simulink model "FullSystem"  (R2024a)
settings: Solver=VariableStepAuto  StartTime=0.0  StopTime=14*3600  RelTol=1e-3
undefined symbols (not defined in the file or in its folder): Beta, D_eq_Linear, GearRatio, I_eq_NonLinear, I_motor, I_Pole, k_b, k_t, L_Motor, Length_Panel, Mass_Panel, R_Motor, StartingPosition, TF_Denom_2, TF_Denom_3, TF_Num_2, TF_Num_3, Thickness_Panel, Width_Panel
libraries: simulink x14, slpidlib x3, slctrl_linear x1
settings Model: Creator=jonat  LastModifiedBy=jonat
settings DataIOCC: ExternalInput=[sunTime,sunPos]  LoadExternalInput=on

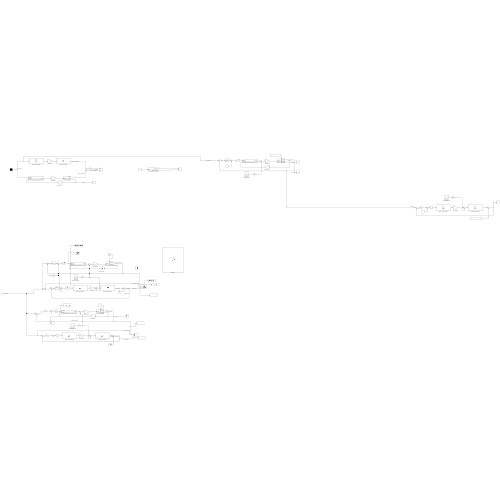
[thumbnail: Simulink's stored preview of the top-level diagram]
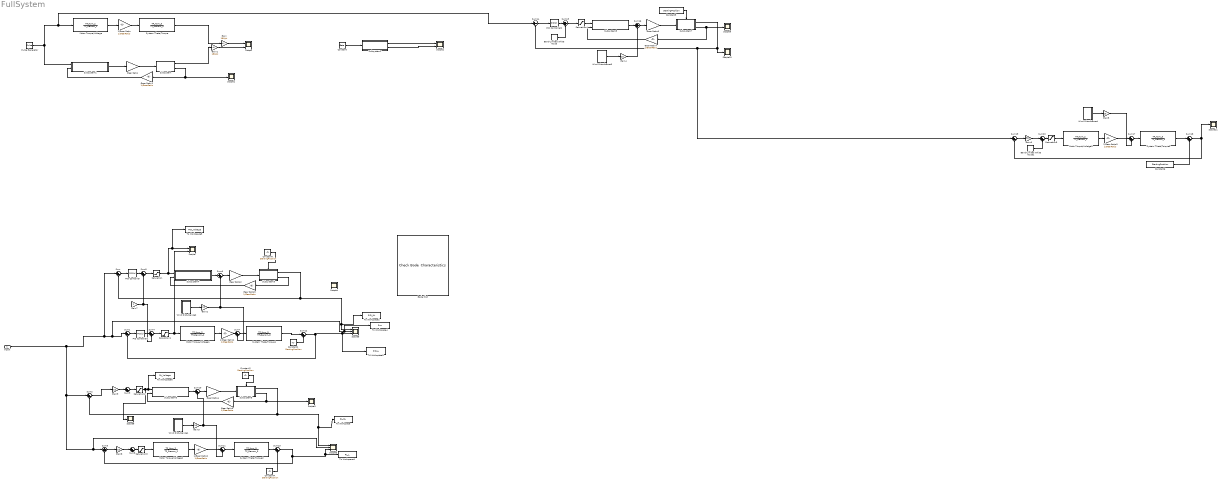
== system FullSystem ==
  Inport : Inport
  1/Gear Ratio{,1..3} (4 alike) : Gain  Gain=1/GearRatio
  Band-Limited White Noise : simulink/Sources/Band-Limited White Noise  Cov=[0.1]  Ts=0.1  seed=[23341]
  Band-Limited White Noise1 : simulink/Sources/Band-Limited White Noise  Cov=[0.1]  Ts=0.1  seed=[23341]
  Bode Plot : slctrl_linear/Check Bode  Characteristics  InstantiateOnLoad=on  SaveOperatingPoints=off  LinearizationIOs={'/PID Controller', 1, 'in', 'off', '';'/Subsystem3', 1, 'out', 'off', ''}  LinearizeAt=SnapshotTimes  SnapshotTimes=[0]  TriggerType=rising  SampleTime=auto  RateConversionMethod=zoh  PreWarpFreq=10  UseExactDelayModel=off  UseFullBlockNameLabels=off  UseBusSignalLabels=off  enabled=on  stopWhenAssertionFail=off  export=off  ViewDlgPos=[345 171 1226 663]  OpenViewOnLoad=off  LaunchViewOnOpen=on  FrequencyUnits=rad/s  MagnitudeUnits=dB  PhaseUnits=deg  TimeUnits=seconds  EnableUpperBound=off  UpperBoundFrequencies=[]  UpperBoundMagnitudes=[]  EnableLowerBound=off  LowerBoundFrequencies=[]  LowerBoundMagnitudes=[]
      settings: LibrarySourceBlock=slctrlblks/Linear Analysis Plots/Bode Plot  SaveToWorkspace=off  SaveName=sys
  Constant : Constant  Value=Beta
  Constant{1..6} (6 alike) : Constant  Value=StartingPosition
  Gain : Gain  Gain=180/pi
  Gain1 : Gain  Gain=180/pi
  Gain{2..5} (4 alike) : Gain  Gain=10
  Gain6 : Gain  Gain=910
  Gain7 : Gain
  Gain8 : Gain  Gain=910
  Gain9 : Gain  Gain=910
  Gear Ratio{,2,4,6} (4 alike) : Gain  Gain=GearRatio
  Gear Ratio{1,3,5,7} (4 alike) : Gain  Gain=1/GearRatio
  Motor Torque/Voltage{,1..3} (4 alike) : TransferFcn  Numerator=TF_Num_2  Denominator=TF_Denom_2
  PID Controller : slpidlib/PID Controller  Controller=PID  Form=Parallel  TimeDomain=Continuous-time  UseExternalTs=off  SampleTime=-1  IntegratorMethod=Forward Euler  FilterMethod=Forward Euler  ControllerParametersSource=internal  P=900  I=2  UseKiTs=off  D=0.1  UseExternalDerivativeSource=off  N=100  UseFilter=on  TunerSelectOption=Transfer Function Based (PID Tuner App)  InitialConditionSource=internal  InitialConditionForIntegrator=0  InitialConditionForFilter=0  DifferentiatorICPrevScaledInput=0  ExternalReset=none  TrackingMode=off  Kt=1  LimitOutput=off  SatLimitsSource=internal  UpperSaturationLimit=inf  LowerSaturationLimit=-inf  LinearizeAsGain=on  AntiWindupMode=none  Kb=1  LimitIntegrator=off  UpperIntegratorSaturationLimit=inf  LowerIntegratorSaturationLimit=-inf  POutMin=[]  POutMax=[]  IOutMin=[]  IOutMax=[]  DOutMin=[]  DOutMax=[]  NOutMin=[]  NOutMax=[]  SumOutMin=[]  SumOutMax=[]  SaturationOutMin=[]  SaturationOutMax=[]  PParamMin=[]  PParamMax=[]  IParamMin=[]  IParamMax=[]  DParamMin=[]  DParamMax=[]  NParamMin=[]  NParamMax=[]  KbParamMin=[]  KbParamMax=[]  KtParamMin=[]  KtParamMax=[]  KbOutMin=[]  KbOutMax=[]  KtOutMin=[]  KtOutMax=[]  IntegratorOutMin=[]  IntegratorOutMax=[]  FilterOutMin=[]  FilterOutMax=[]  SumI1OutMin=[]  SumI1OutMax=[]  SumI2OutMin=[]  SumI2OutMax=[]  SumI3OutMin=[]  SumI3OutMax=[]  SumI4OutMin=[]  SumI4OutMax=[]  SumDOutMin=[]  SumDOutMax=[]  DifferentiatorOutMin=[]  DifferentiatorOutMax=[]  FilterDiffOutCoefMin=[]  FilterDiffOutCoefMax=[]  ReciprocalOutMin=[]  ReciprocalOutMax=[]  SumDenOutMin=[]  SumDenOutMax=[]  SumNumOutMin=[]  SumNumOutMax=[]  DivideOutMin=[]  DivideOutMax=[]  UdiffTsProdOutMin=[]  UdiffTsProdOutMax=[]  NTsProdOutMin=[]  NTsProdOutMax=[]  UintegralTsProdOutMin=[]  UintegralTsProdOutMax=[]  UngainTsProdOutMin=[]  UngainTsProdOutMax=[]  ClampingZeroOutDataTypeStr=Inherit: Inherit via back propagation  ClampingZeroOutMin=[]  ClampingZeroOutMax=[]  FilterDenConstantOutDataTypeStr=Inherit: Inherit via back propagation  FilterDenConstantOutMin=[]  FilterDenConstantOutMax=[]  PCopyOutDataTypeStr=Inherit: Inherit via back propagation  PCopyOutMin=[]  PCopyOutMax=[]  NCopyOutDataTypeStr=Inherit: Inherit via back propagation  NCopyOutMin=[]  NCopyOutMax=[]  IntegratorContinuousStateAttributes=''  IntegratorStateMustResolveToSignalObject=off  IntegratorRTWStateStorageClass=Auto  FilterContinuousStateAttributes=''  FilterStateMustResolveToSignalObject=off  FilterRTWStateStorageClass=Auto  ParallelPVariant=InternalParameters  IdealPVariant=Disabled  IVariant=InternalParameters  DVariant=InternalParameters  IntegratorVariant=Continuous  SatVariant=Disabled  AWVariant=Passthrough  PCopyVariant=Disabled  TRVariant=Disabled  FdbkBlocksVariant=Forward  IdealPFdbkVariant=Disabled  SatFdbkVariant=Disabled  DerivativeFilterVariant=ContFilter  NVariant=InternalParameters  NCopyVariant=Disabled  FilterICVariant=InternalICsFilter  IntegratorICVariant=InternalICs  ExternalResetVariant=Disabled  TRSumVariant=Passthrough  SumFdbkVariant=Disabled  SumVariant=Sum_PID  TsampFilterVariant=InternalTs  TsampNgainVariant=Passthrough  TsampIntegralVariant=Disabled_SignalSpec  ExternalSaturationOutDataTypeStr=Inherit: Same as second input  DerivativeSourceVariant=ErrorSignal
  PID Controller1 : slpidlib/PID Controller  Controller=PID  Form=Parallel  TimeDomain=Continuous-time  UseExternalTs=off  SampleTime=-1  IntegratorMethod=Forward Euler  FilterMethod=Forward Euler  ControllerParametersSource=internal  P=900  I=2  UseKiTs=off  D=0.1  UseExternalDerivativeSource=off  N=2.09794311620465  UseFilter=on  TunerSelectOption=Transfer Function Based (PID Tuner App)  InitialConditionSource=internal  InitialConditionForIntegrator=0  InitialConditionForFilter=0  DifferentiatorICPrevScaledInput=0  ExternalReset=none  TrackingMode=off  Kt=1  LimitOutput=off  SatLimitsSource=internal  UpperSaturationLimit=inf  LowerSaturationLimit=-inf  LinearizeAsGain=on  AntiWindupMode=none  Kb=1  LimitIntegrator=off  UpperIntegratorSaturationLimit=inf  LowerIntegratorSaturationLimit=-inf  POutMin=[]  POutMax=[]  IOutMin=[]  IOutMax=[]  DOutMin=[]  DOutMax=[]  NOutMin=[]  NOutMax=[]  SumOutMin=[]  SumOutMax=[]  SaturationOutMin=[]  SaturationOutMax=[]  PParamMin=[]  PParamMax=[]  IParamMin=[]  IParamMax=[]  DParamMin=[]  DParamMax=[]  NParamMin=[]  NParamMax=[]  KbParamMin=[]  KbParamMax=[]  KtParamMin=[]  KtParamMax=[]  KbOutMin=[]  KbOutMax=[]  KtOutMin=[]  KtOutMax=[]  IntegratorOutMin=[]  IntegratorOutMax=[]  FilterOutMin=[]  FilterOutMax=[]  SumI1OutMin=[]  SumI1OutMax=[]  SumI2OutMin=[]  SumI2OutMax=[]  SumI3OutMin=[]  SumI3OutMax=[]  SumI4OutMin=[]  SumI4OutMax=[]  SumDOutMin=[]  SumDOutMax=[]  DifferentiatorOutMin=[]  DifferentiatorOutMax=[]  FilterDiffOutCoefMin=[]  FilterDiffOutCoefMax=[]  ReciprocalOutMin=[]  ReciprocalOutMax=[]  SumDenOutMin=[]  SumDenOutMax=[]  SumNumOutMin=[]  SumNumOutMax=[]  DivideOutMin=[]  DivideOutMax=[]  UdiffTsProdOutMin=[]  UdiffTsProdOutMax=[]  NTsProdOutMin=[]  NTsProdOutMax=[]  UintegralTsProdOutMin=[]  UintegralTsProdOutMax=[]  UngainTsProdOutMin=[]  UngainTsProdOutMax=[]  ClampingZeroOutDataTypeStr=Inherit: Inherit via back propagation  ClampingZeroOutMin=[]  ClampingZeroOutMax=[]  FilterDenConstantOutDataTypeStr=Inherit: Inherit via back propagation  FilterDenConstantOutMin=[]  FilterDenConstantOutMax=[]  PCopyOutDataTypeStr=Inherit: Inherit via back propagation  PCopyOutMin=[]  PCopyOutMax=[]  NCopyOutDataTypeStr=Inherit: Inherit via back propagation  NCopyOutMin=[]  NCopyOutMax=[]  IntegratorContinuousStateAttributes=''  IntegratorStateMustResolveToSignalObject=off  IntegratorRTWStateStorageClass=Auto  FilterContinuousStateAttributes=''  FilterStateMustResolveToSignalObject=off  FilterRTWStateStorageClass=Auto  ParallelPVariant=InternalParameters  IdealPVariant=Disabled  IVariant=InternalParameters  DVariant=InternalParameters  IntegratorVariant=Continuous  SatVariant=Disabled  AWVariant=Passthrough  PCopyVariant=Disabled  TRVariant=Disabled  FdbkBlocksVariant=Forward  IdealPFdbkVariant=Disabled  SatFdbkVariant=Disabled  DerivativeFilterVariant=ContFilter  NVariant=InternalParameters  NCopyVariant=Disabled  FilterICVariant=InternalICsFilter  IntegratorICVariant=InternalICs  ExternalResetVariant=Disabled  TRSumVariant=Passthrough  SumFdbkVariant=Disabled  SumVariant=Sum_PID  TsampFilterVariant=InternalTs  TsampNgainVariant=Passthrough  TsampIntegralVariant=Disabled_SignalSpec  ExternalSaturationOutDataTypeStr=Inherit: Same as second input  DerivativeSourceVariant=ErrorSignal
  PID Controller2 : slpidlib/PID Controller  Controller=PID  Form=Parallel  TimeDomain=Continuous-time  UseExternalTs=off  SampleTime=-1  IntegratorMethod=Forward Euler  FilterMethod=Forward Euler  ControllerParametersSource=internal  P=900  I=2  UseKiTs=off  D=0.1  UseExternalDerivativeSource=off  N=100  UseFilter=on  TunerSelectOption=Transfer Function Based (PID Tuner App)  InitialConditionSource=internal  InitialConditionForIntegrator=0  InitialConditionForFilter=0  DifferentiatorICPrevScaledInput=0  ExternalReset=none  TrackingMode=off  Kt=1  LimitOutput=off  SatLimitsSource=internal  UpperSaturationLimit=inf  LowerSaturationLimit=-inf  LinearizeAsGain=on  AntiWindupMode=none  Kb=1  LimitIntegrator=off  UpperIntegratorSaturationLimit=inf  LowerIntegratorSaturationLimit=-inf  POutMin=[]  POutMax=[]  IOutMin=[]  IOutMax=[]  DOutMin=[]  DOutMax=[]  NOutMin=[]  NOutMax=[]  SumOutMin=[]  SumOutMax=[]  SaturationOutMin=[]  SaturationOutMax=[]  PParamMin=[]  PParamMax=[]  IParamMin=[]  IParamMax=[]  DParamMin=[]  DParamMax=[]  NParamMin=[]  NParamMax=[]  KbParamMin=[]  KbParamMax=[]  KtParamMin=[]  KtParamMax=[]  KbOutMin=[]  KbOutMax=[]  KtOutMin=[]  KtOutMax=[]  IntegratorOutMin=[]  IntegratorOutMax=[]  FilterOutMin=[]  FilterOutMax=[]  SumI1OutMin=[]  SumI1OutMax=[]  SumI2OutMin=[]  SumI2OutMax=[]  SumI3OutMin=[]  SumI3OutMax=[]  SumI4OutMin=[]  SumI4OutMax=[]  SumDOutMin=[]  SumDOutMax=[]  DifferentiatorOutMin=[]  DifferentiatorOutMax=[]  FilterDiffOutCoefMin=[]  FilterDiffOutCoefMax=[]  ReciprocalOutMin=[]  ReciprocalOutMax=[]  SumDenOutMin=[]  SumDenOutMax=[]  SumNumOutMin=[]  SumNumOutMax=[]  DivideOutMin=[]  DivideOutMax=[]  UdiffTsProdOutMin=[]  UdiffTsProdOutMax=[]  NTsProdOutMin=[]  NTsProdOutMax=[]  UintegralTsProdOutMin=[]  UintegralTsProdOutMax=[]  UngainTsProdOutMin=[]  UngainTsProdOutMax=[]  ClampingZeroOutDataTypeStr=Inherit: Inherit via back propagation  ClampingZeroOutMin=[]  ClampingZeroOutMax=[]  FilterDenConstantOutDataTypeStr=Inherit: Inherit via back propagation  FilterDenConstantOutMin=[]  FilterDenConstantOutMax=[]  PCopyOutDataTypeStr=Inherit: Inherit via back propagation  PCopyOutMin=[]  PCopyOutMax=[]  NCopyOutDataTypeStr=Inherit: Inherit via back propagation  NCopyOutMin=[]  NCopyOutMax=[]  IntegratorContinuousStateAttributes=''  IntegratorStateMustResolveToSignalObject=off  IntegratorRTWStateStorageClass=Auto  FilterContinuousStateAttributes=''  FilterStateMustResolveToSignalObject=off  FilterRTWStateStorageClass=Auto  ParallelPVariant=InternalParameters  IdealPVariant=Disabled  IVariant=InternalParameters  DVariant=InternalParameters  IntegratorVariant=Continuous  SatVariant=Disabled  AWVariant=Passthrough  PCopyVariant=Disabled  TRVariant=Disabled  FdbkBlocksVariant=Forward  IdealPFdbkVariant=Disabled  SatFdbkVariant=Disabled  DerivativeFilterVariant=ContFilter  NVariant=InternalParameters  NCopyVariant=Disabled  FilterICVariant=InternalICsFilter  IntegratorICVariant=InternalICs  ExternalResetVariant=Disabled  TRSumVariant=Passthrough  SumFdbkVariant=Disabled  SumVariant=Sum_PID  TsampFilterVariant=InternalTs  TsampNgainVariant=Passthrough  TsampIntegralVariant=Disabled_SignalSpec  ExternalSaturationOutDataTypeStr=Inherit: Same as second input  DerivativeSourceVariant=ErrorSignal
  Pulse Generator : DiscretePulseGenerator  PulseType=Time based  Amplitude=5  Period=400
  Saturation{,1..5} (6 alike) : Saturate  UpperLimit=220  LowerLimit=-220
  Scope : Scope  NumInputPorts=2
  Scope{1,3..4,8..11} (7 alike) : Scope
  Scope2 : Scope  NumInputPorts=2
  Scope5 : Scope  NumInputPorts=3
  Scope6 : Scope  NumInputPorts=3
  Scope7 : Scope  NumInputPorts=2
  Subsystem : Subsystem
  Subsystem1 : Subsystem
  Subsystem2 : Subsystem
  Subsystem3 : Subsystem
      settings: PortSchema="{\"entries\":[{\"content\":{\"sides\":[{\"content\":{\"connectorIds\":[\"In1\"]},\"type\":\"ConnectorPlacement.EquallySpacedRectSide\",\"uuid\":\"8ea1f8af-770d-4a24-b012-ba6e01ad0303\"},{\"content\":{\"connectorIds\":[\"Out1\",\"Out2\"],\"side\":\"RIGHT\"},\"type\":\"ConnectorPlacement.EquallySpacedRectSide\",\"uuid\":\"5c008235-f776-4735-b061-be577f1b76a0\"},{\"content\":{\"connectorIds\":[\"In2\"],\"side\":\"TOP\"},\"type\":\"ConnectorPlacement.EquallySpacedRectSide\",\"uuid\":\"8e8587eb-de19-4631-a42c-bfa0ae223d11\"}]},\"type\":\"ConnectorPlacement.EquallySpacedConnector\",\"uuid\":\"de8c275b-bedc-409d-bb08-97ede13c9c40\"}],\"packageUris\":[\"http://schema.mathworks.com/mf0/Connector/R2020b\"],\"version\":\"1.0\"}"
  Subsystem4 : Subsystem
  Subsystem5 : Subsystem
      settings: PortSchema="{\"entries\":[{\"content\":{\"sides\":[{\"content\":{\"connectorIds\":[\"In1\"]},\"type\":\"ConnectorPlacement.EquallySpacedRectSide\",\"uuid\":\"8ea1f8af-770d-4a24-b012-ba6e01ad0303\"},{\"content\":{\"connectorIds\":[\"Out1\",\"Out2\"],\"side\":\"RIGHT\"},\"type\":\"ConnectorPlacement.EquallySpacedRectSide\",\"uuid\":\"5c008235-f776-4735-b061-be577f1b76a0\"},{\"content\":{\"connectorIds\":[\"In2\"],\"side\":\"TOP\"},\"type\":\"ConnectorPlacement.EquallySpacedRectSide\",\"uuid\":\"8e8587eb-de19-4631-a42c-bfa0ae223d11\"}]},\"type\":\"ConnectorPlacement.EquallySpacedConnector\",\"uuid\":\"de8c275b-bedc-409d-bb08-97ede13c9c40\"}],\"packageUris\":[\"http://schema.mathworks.com/mf0/Connector/R2020b\"],\"version\":\"1.0\"}"
  Subsystem6 : Subsystem
  Subsystem7 : Subsystem
      settings: PortSchema="{\"entries\":[{\"content\":{\"sides\":[{\"content\":{\"connectorIds\":[\"In1\"]},\"type\":\"ConnectorPlacement.EquallySpacedRectSide\",\"uuid\":\"8ea1f8af-770d-4a24-b012-ba6e01ad0303\"},{\"content\":{\"connectorIds\":[\"Out1\",\"Out2\"],\"side\":\"RIGHT\"},\"type\":\"ConnectorPlacement.EquallySpacedRectSide\",\"uuid\":\"5c008235-f776-4735-b061-be577f1b76a0\"},{\"content\":{\"connectorIds\":[\"In2\"],\"side\":\"TOP\"},\"type\":\"ConnectorPlacement.EquallySpacedRectSide\",\"uuid\":\"8e8587eb-de19-4631-a42c-bfa0ae223d11\"}]},\"type\":\"ConnectorPlacement.EquallySpacedConnector\",\"uuid\":\"de8c275b-bedc-409d-bb08-97ede13c9c40\"}],\"packageUris\":[\"http://schema.mathworks.com/mf0/Connector/R2020b\"],\"version\":\"1.0\"}"
  Subsystem8 : Subsystem
  Sum{,1..3,14,19} (6 alike) : Sum  Inputs=|+-
  Sum{4..13,15..18,20} (15 alike) : Sum  Inputs=|++
  System Theta/Torque{,1..3} (4 alike) : TransferFcn  Numerator=TF_Num_3  Denominator=TF_Denom_3
  To Workspace : ToWorkspace  VariableName=RL_NL  SampleTime=-1
  To Workspace1 : ToWorkspace  VariableName=RL_L  SampleTime=-1
  To Workspace2 : ToWorkspace  VariableName=PID_NL  SampleTime=-1
  To Workspace3 : ToWorkspace  VariableName=PID_L  SampleTime=-1
  To Workspace4 : ToWorkspace  VariableName=Sun  SampleTime=-1
  To Workspace5 : ToWorkspace  VariableName=PID_Voltage  SampleTime=-1
  To Workspace6 : ToWorkspace  VariableName=RL_Voltage  SampleTime=-1
  Wind Disturbance1 : Subsystem
  Wind Disturbance2 : Subsystem
  Wind Disturbance3 : Subsystem
  Wind Disturbance4 : Subsystem
  wires:
  Subsystem/1(Position) -> Gain1/1  "Position Non-Linear"
  Subsystem/2(Velocity) -> Gear Ratio1/1, Scope1/1  "Velocity"
  Subsystem1/1(Torque) -> Gear Ratio/1
  Gear Ratio/1 -> Subsystem/1(Torque)
  1/Gear Ratio/1 -> System Theta/Torque/1
  Motor Torque/Voltage/1 -> 1/Gear Ratio/1
  System Theta/Torque/1 -> Gain/1  "Position Linear Model"
  Gear Ratio1/1 -> Subsystem1/2(Velocity)
  Constant/1 -> Subsystem2/1(Beta)
  Subsystem2/1(MOI Linear) -> Scope2/1
  Subsystem2/2(MOI Non Linear) -> Scope2/2
  Gain/1 -> Scope/1  "Linear Model"
  Gain1/1 -> Scope/2  "Non-Linear Model"
  Subsystem3/1(Position) -> Scope5/1, To Workspace2/1, Sum/2  "Position Non-Linear"
  Subsystem4/1(Torque) -> Sum6/1
  Gear Ratio2/1 -> Subsystem3/1(Torque)
  Subsystem3/2(Velocity) -> Gear Ratio3/1  "Velocity"
  Gear Ratio3/1 -> Subsystem4/2(Velocity)
  Sum/1 -> PID Controller/1  "Error"
  PID Controller/1 -> Sum5/1
  Motor Torque/Voltage1/1 -> 1/Gear Ratio1/1
  1/Gear Ratio1/1 -> Sum7/1
  PID Controller1/1 -> Sum4/1
  Sum1/1 -> PID Controller1/1  "Error"
  Sum12/1 -> Sum1/2, To Workspace3/1, Scope5/3  "Linear Model"
  1/Gear Ratio2/1 -> Sum11/1
  Motor Torque/Voltage2/1 -> 1/Gear Ratio2/1
  Subsystem6/1(Torque) -> Sum10/1
  Sum2/1 -> Gain9/1  "Error"
  Gear Ratio5/1 -> Subsystem6/2(Velocity)
  Gear Ratio4/1 -> Subsystem5/1(Torque)
  Sum3/1 -> Gain8/1  "Error"
  Subsystem5/2(Velocity) -> Gear Ratio5/1, Scope3/1  "Velocity"
  Subsystem5/1(Position) -> Sum2/2, Scope6/1, To Workspace/1  "Position Non-Linear"
  Sum4/1 -> Saturation1/1
  Sum13/1 -> To Workspace1/1, Scope6/3, Sum3/2  "Linear Model"
  Gain8/1 -> Sum8/1
  Gain9/1 -> Sum9/1
  Inport/1 -> Sum2/1, Scope6/2, Sum3/1, Sum/1, To Workspace4/1, Scope5/2, Sum1/1  "Sun Positon"
  Sum6/1 -> Gear Ratio2/1
  Sum7/1 -> System Theta/Torque1/1
  Sum9/1 -> Saturation2/1
  Sum10/1 -> Gear Ratio4/1
  Sum11/1 -> System Theta/Torque2/1
  Gain3/1 -> Sum11/2, Sum10/2
  Gain2/1 -> Sum7/2, Sum6/2
  Wind Disturbance1/1(Out1) -> Gain3/1
  System Theta/Torque1/1 -> Sum12/1  "Linear Model"
  Constant1/1 -> Sum12/2
  Sum5/1 -> Saturation/1
  Saturation/1 -> Subsystem4/1(Voltage), To Workspace5/1, Scope7/1
  Constant2/1 -> Subsystem3/2(StartPos)
  Constant3/1 -> Subsystem5/2(StartPosRL)
  System Theta/Torque2/1 -> Sum13/1  "Linear Model"
  Constant4/1 -> Sum13/2
  Saturation1/1 -> Scope7/2, Motor Torque/Voltage1/1
  Saturation2/1 -> Scope8/1, To Workspace6/1, Subsystem6/1(Voltage)
  Sum8/1 -> Saturation3/1
  Saturation3/1 -> Motor Torque/Voltage2/1
  Gain7/1 -> Sum4/2, Sum5/2
  Band-Limited White Noise/1 -> Sum15/2
  Saturation4/1 -> Subsystem8/1(Voltage)
  Subsystem7/2(Velocity) -> Gear Ratio7/1, Scope9/1  "Velocity"
  Pulse Generator/1 -> Sum14/1, Motor Torque/Voltage/1, Subsystem1/1(Voltage)  "Sun Positon"
  Constant5/1 -> Subsystem7/2(StartPos)
  Gain4/1 -> Sum16/2
  Sum14/1 -> PID Controller2/1  "Error"
  Sum15/1 -> Saturation4/1
  Gear Ratio6/1 -> Subsystem7/1(Torque)
  Wind Disturbance3/1(Out1) -> Gain4/1
  Sum16/1 -> Gear Ratio6/1
  Gear Ratio7/1 -> Subsystem8/2(Velocity)
  PID Controller2/1 -> Sum15/1
  Subsystem8/1(Torque) -> Sum16/1
  System Theta/Torque3/1 -> Sum18/1
  Sum20/1 -> Saturation5/1
  Saturation5/1 -> Motor Torque/Voltage3/1
  Constant6/1 -> Sum18/2
  Sum17/1 -> System Theta/Torque3/1
  Sum18/1 -> Sum19/2, Scope11/1
  Gain5/1 -> Sum17/2
  Gain6/1 -> Sum20/1
  Subsystem7/1(Position) -> Sum19/1, Sum14/2, Scope10/1  "Sun Positon"
  1/Gear Ratio3/1 -> Sum17/1
  Motor Torque/Voltage3/1 -> 1/Gear Ratio3/1
  Sum19/1 -> Gain6/1  "Error"
  Wind Disturbance4/1(Out1) -> Gain5/1
  Band-Limited White Noise1/1 -> Sum20/2
  ? -> Gain7/1
  Wind Disturbance2/1(Out1) -> Gain2/1

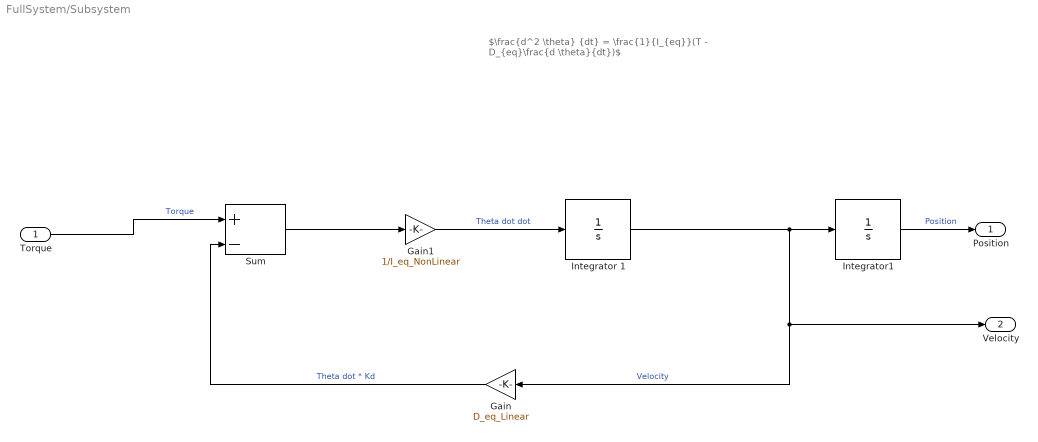
== system FullSystem/Subsystem ==
  note: $\frac{d^2 \theta} {dt} = \frac{1}{I_{eq}}(T - D_{eq}\frac{d \theta}{dt})$
  Torque : Inport
  Gain : Gain  Gain=D_eq_Linear
  Gain1 : Gain  Gain=1/I_eq_NonLinear
  Integrator 1 : Integrator
  Integrator1 : Integrator
  Sum : Sum  Inputs=|+-
  Position : Outport
  Velocity : Outport  Port=2
  wires:
  Sum/1 -> Gain1/1
  Integrator1/1 -> Position/1  "Position"
  Gain1/1 -> Integrator 1/1  "Theta dot dot"
  Integrator 1/1 -> Velocity/1, Gain/1, Integrator1/1  "Velocity"
  Torque/1 -> Sum/1  "Torque"
  Gain/1 -> Sum/2  "Theta dot * Kd"

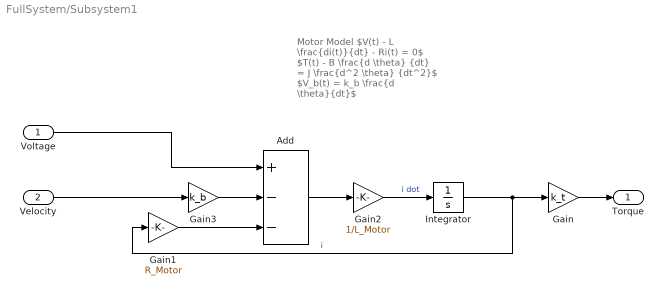
== system FullSystem/Subsystem1 ==
  note: Motor Model
      | $V(t) - L \frac{di(t)}{dt} - Ri(t) = 0$
      | $T(t) - B \frac{d \theta} {dt} = J \frac{d^2 \theta} {dt^2}$
      | $V_b(t) = k_b \frac{d \theta}{dt}$
  Voltage : Inport
  Velocity : Inport  Port=2
  Add : Sum  Inputs=+--
  Gain : Gain  Gain=k_t
  Gain1 : Gain  Gain=R_Motor
  Gain2 : Gain  Gain=1/L_Motor
  Gain3 : Gain  Gain=k_b
  Integrator : Integrator
  Torque : Outport
  wires:
  Integrator/1 -> Gain/1, Gain1/1  "i"
  Add/1 -> Gain2/1
  Gain3/1 -> Add/2
  Velocity/1 -> Gain3/1
  Voltage/1 -> Add/1
  Gain/1 -> Torque/1
  Gain2/1 -> Integrator/1  "i dot"
  Gain1/1 -> Add/3

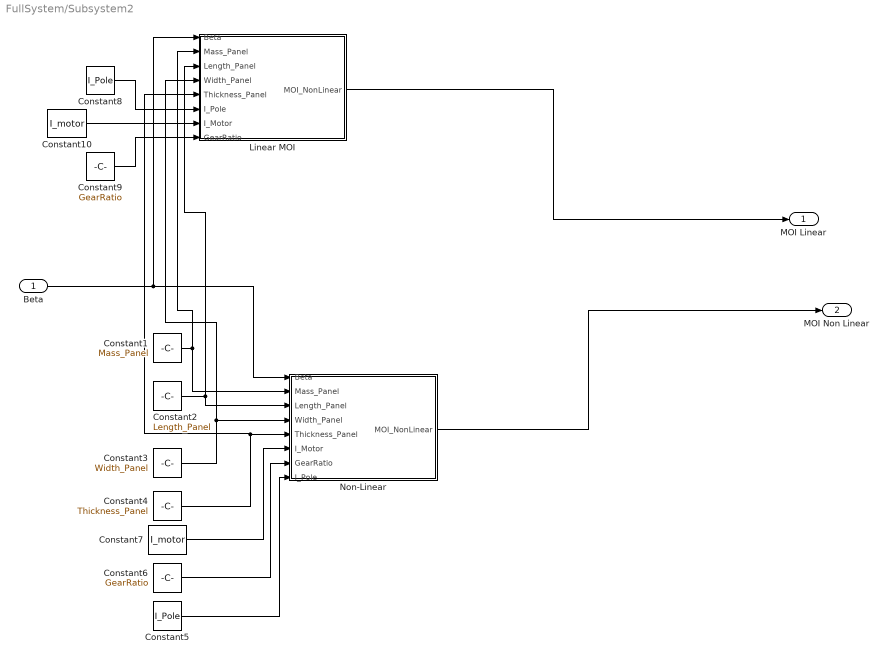
== system FullSystem/Subsystem2 ==
  Beta : Inport
  Constant1 : Constant  Value=Mass_Panel
  Constant10 : Constant  Value=I_motor
  Constant2 : Constant  Value=Length_Panel
  Constant3 : Constant  Value=Width_Panel
  Constant4 : Constant  Value=Thickness_Panel
  Constant5 : Constant  Value=I_Pole
  Constant6 : Constant  Value=GearRatio
  Constant7 : Constant  Value=I_motor
  Constant8 : Constant  Value=I_Pole
  Constant9 : Constant  Value=GearRatio
  Linear MOI : MATLAB Function  TreatAsAtomicUnit=on
  Non-Linear : MATLAB Function  TreatAsAtomicUnit=on
  MOI Linear : Outport
  MOI Non Linear : Outport  Port=2
  wires:
  Constant2/1 -> Linear MOI/3(Length_Panel), Non-Linear/3(Length_Panel)
  Constant6/1 -> Non-Linear/7(GearRatio)
  Constant8/1 -> Linear MOI/6(I_Pole)
  Constant3/1 -> Non-Linear/4(Width_Panel), Linear MOI/4(Width_Panel)
  Constant4/1 -> Non-Linear/5(Thickness_Panel), Linear MOI/5(Thickness_Panel)
  Beta/1 -> Linear MOI/1(Beta), Non-Linear/1(Beta)
  Constant1/1 -> Linear MOI/2(Mass_Panel), Non-Linear/2(Mass_Panel)
  Constant10/1 -> Linear MOI/7(I_Motor)
  Constant7/1 -> Non-Linear/6(I_Motor)
  Constant9/1 -> Linear MOI/8(GearRatio)
  Constant5/1 -> Non-Linear/8(I_Pole)
  Non-Linear/1(MOI_NonLinear) -> MOI Non Linear/1
  Linear MOI/1(MOI_NonLinear) -> MOI Linear/1

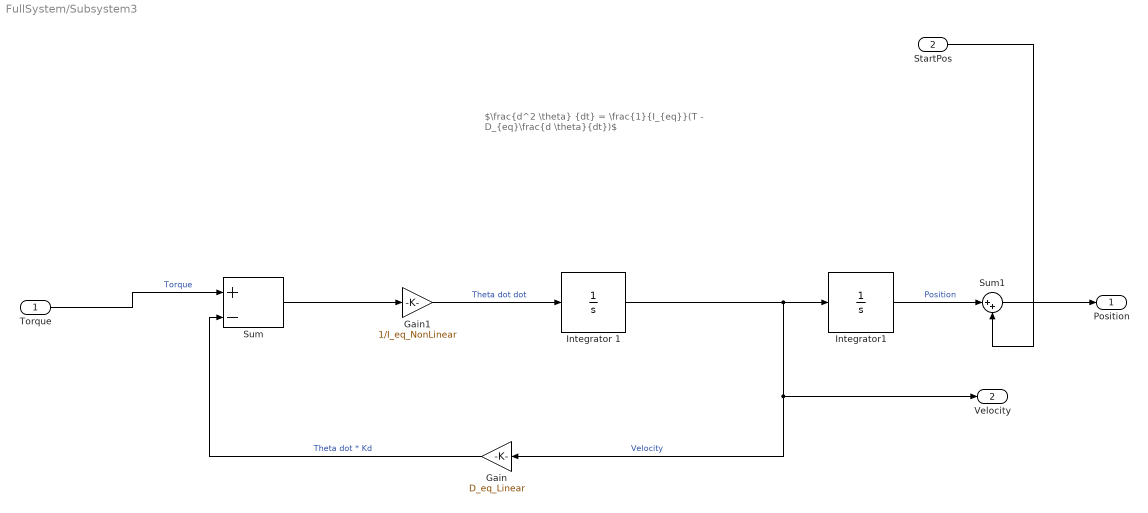
== system FullSystem/Subsystem3 ==
  note: $\frac{d^2 \theta} {dt} = \frac{1}{I_{eq}}(T - D_{eq}\frac{d \theta}{dt})$
  Torque : Inport
  StartPos : Inport  Port=2
  Gain : Gain  Gain=D_eq_Linear
  Gain1 : Gain  Gain=1/I_eq_NonLinear
  Integrator 1 : Integrator
  Integrator1 : Integrator
  Sum : Sum  Inputs=|+-
  Sum1 : Sum  Inputs=|++
  Position : Outport
  Velocity : Outport  Port=2
  wires:
  Sum/1 -> Gain1/1
  Integrator1/1 -> Sum1/1  "Position"
  Gain1/1 -> Integrator 1/1  "Theta dot dot"
  Integrator 1/1 -> Velocity/1, Gain/1, Integrator1/1  "Velocity"
  Torque/1 -> Sum/1  "Torque"
  Gain/1 -> Sum/2  "Theta dot * Kd"
  Sum1/1 -> Position/1
  StartPos/1 -> Sum1/2

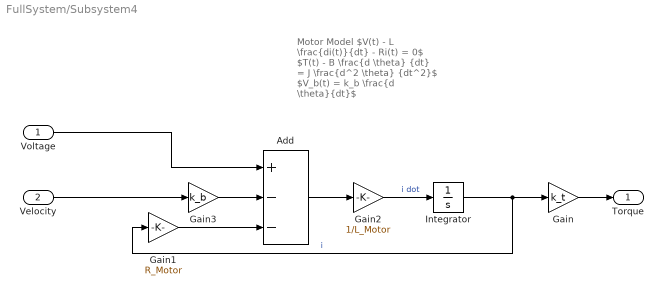
== system FullSystem/Subsystem4 ==
  note: Motor Model
      | $V(t) - L \frac{di(t)}{dt} - Ri(t) = 0$
      | $T(t) - B \frac{d \theta} {dt} = J \frac{d^2 \theta} {dt^2}$
      | $V_b(t) = k_b \frac{d \theta}{dt}$
  Voltage : Inport
  Velocity : Inport  Port=2
  Add : Sum  Inputs=+--
  Gain : Gain  Gain=k_t
  Gain1 : Gain  Gain=R_Motor
  Gain2 : Gain  Gain=1/L_Motor
  Gain3 : Gain  Gain=k_b
  Integrator : Integrator
  Torque : Outport
  wires:
  Integrator/1 -> Gain/1, Gain1/1  "i"
  Add/1 -> Gain2/1
  Gain3/1 -> Add/2
  Velocity/1 -> Gain3/1
  Voltage/1 -> Add/1
  Gain/1 -> Torque/1
  Gain2/1 -> Integrator/1  "i dot"
  Gain1/1 -> Add/3

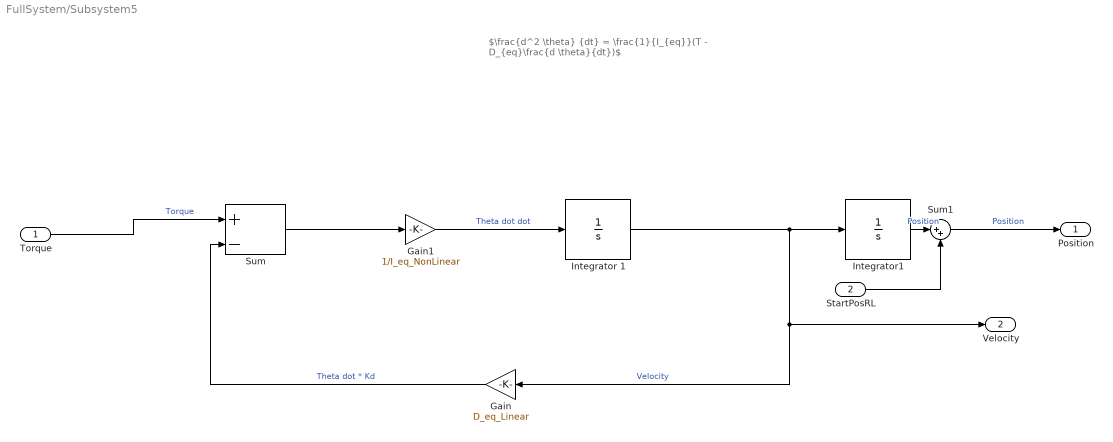
== system FullSystem/Subsystem5 ==
  note: $\frac{d^2 \theta} {dt} = \frac{1}{I_{eq}}(T - D_{eq}\frac{d \theta}{dt})$
  Torque : Inport
  StartPosRL : Inport  Port=2
  Gain : Gain  Gain=D_eq_Linear
  Gain1 : Gain  Gain=1/I_eq_NonLinear
  Integrator 1 : Integrator
  Integrator1 : Integrator
  Sum : Sum  Inputs=|+-
  Sum1 : Sum  Inputs=|++
  Position : Outport
  Velocity : Outport  Port=2
  wires:
  Sum/1 -> Gain1/1
  Sum1/1 -> Position/1  "Position"
  Gain1/1 -> Integrator 1/1  "Theta dot dot"
  Integrator 1/1 -> Velocity/1, Gain/1, Integrator1/1  "Velocity"
  Torque/1 -> Sum/1  "Torque"
  Gain/1 -> Sum/2  "Theta dot * Kd"
  Integrator1/1 -> Sum1/1  "Position"
  StartPosRL/1 -> Sum1/2

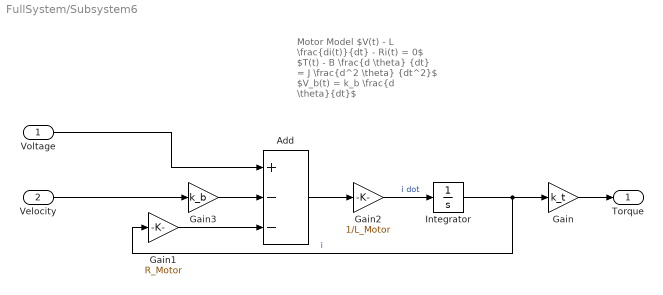
== system FullSystem/Subsystem6 ==
  note: Motor Model
      | $V(t) - L \frac{di(t)}{dt} - Ri(t) = 0$
      | $T(t) - B \frac{d \theta} {dt} = J \frac{d^2 \theta} {dt^2}$
      | $V_b(t) = k_b \frac{d \theta}{dt}$
  Voltage : Inport
  Velocity : Inport  Port=2
  Add : Sum  Inputs=+--
  Gain : Gain  Gain=k_t
  Gain1 : Gain  Gain=R_Motor
  Gain2 : Gain  Gain=1/L_Motor
  Gain3 : Gain  Gain=k_b
  Integrator : Integrator
  Torque : Outport
  wires:
  Integrator/1 -> Gain/1, Gain1/1  "i"
  Add/1 -> Gain2/1
  Gain3/1 -> Add/2
  Velocity/1 -> Gain3/1
  Voltage/1 -> Add/1
  Gain/1 -> Torque/1
  Gain2/1 -> Integrator/1  "i dot"
  Gain1/1 -> Add/3

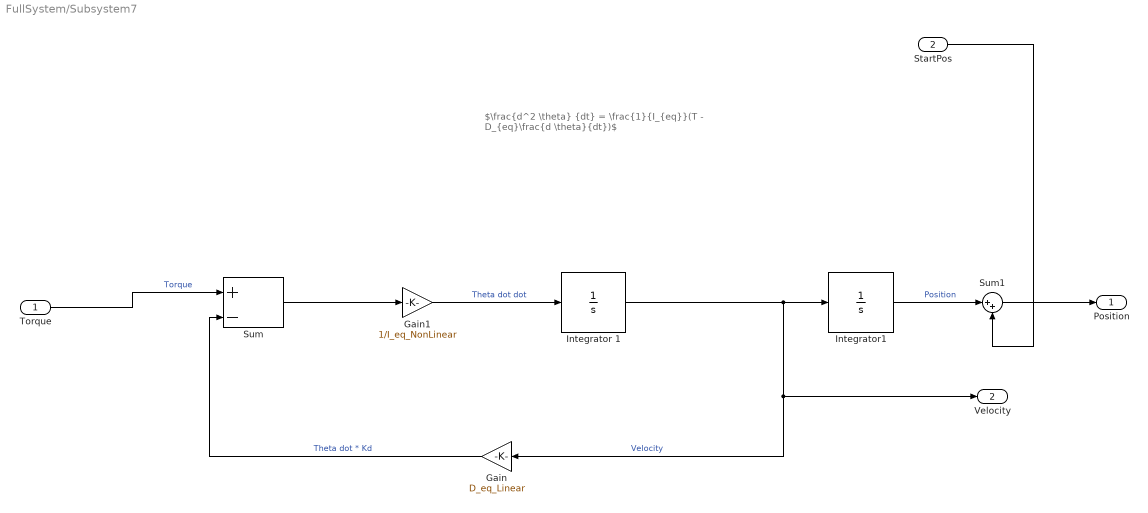
== system FullSystem/Subsystem7 ==
  note: $\frac{d^2 \theta} {dt} = \frac{1}{I_{eq}}(T - D_{eq}\frac{d \theta}{dt})$
  Torque : Inport
  StartPos : Inport  Port=2
  Gain : Gain  Gain=D_eq_Linear
  Gain1 : Gain  Gain=1/I_eq_NonLinear
  Integrator 1 : Integrator
  Integrator1 : Integrator
  Sum : Sum  Inputs=|+-
  Sum1 : Sum  Inputs=|++
  Position : Outport
  Velocity : Outport  Port=2
  wires:
  Sum/1 -> Gain1/1
  Integrator1/1 -> Sum1/1  "Position"
  Gain1/1 -> Integrator 1/1  "Theta dot dot"
  Integrator 1/1 -> Velocity/1, Gain/1, Integrator1/1  "Velocity"
  Torque/1 -> Sum/1  "Torque"
  Gain/1 -> Sum/2  "Theta dot * Kd"
  Sum1/1 -> Position/1
  StartPos/1 -> Sum1/2

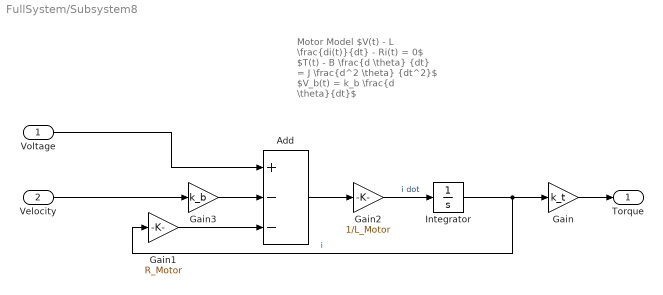
== system FullSystem/Subsystem8 ==
  note: Motor Model
      | $V(t) - L \frac{di(t)}{dt} - Ri(t) = 0$
      | $T(t) - B \frac{d \theta} {dt} = J \frac{d^2 \theta} {dt^2}$
      | $V_b(t) = k_b \frac{d \theta}{dt}$
  Voltage : Inport
  Velocity : Inport  Port=2
  Add : Sum  Inputs=+--
  Gain : Gain  Gain=k_t
  Gain1 : Gain  Gain=R_Motor
  Gain2 : Gain  Gain=1/L_Motor
  Gain3 : Gain  Gain=k_b
  Integrator : Integrator
  Torque : Outport
  wires:
  Integrator/1 -> Gain/1, Gain1/1  "i"
  Add/1 -> Gain2/1
  Gain3/1 -> Add/2
  Velocity/1 -> Gain3/1
  Voltage/1 -> Add/1
  Gain/1 -> Torque/1
  Gain2/1 -> Integrator/1  "i dot"
  Gain1/1 -> Add/3

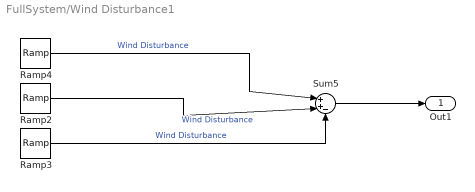
== system FullSystem/Wind Disturbance1 ==
  Ramp2 : simulink/Sources/Ramp  slope=1  start=1000  InitialOutput=0
  Ramp3 : simulink/Sources/Ramp  slope=2  start=1005  InitialOutput=0
  Ramp4 : simulink/Sources/Ramp  slope=1  start=1010  InitialOutput=0
  Sum5 : Sum  Inputs=|++-
  Out1 : Outport
  wires:
  Ramp2/1 -> Sum5/2  "Wind Disturbance"
  Ramp4/1 -> Sum5/1  "Wind Disturbance"
  Sum5/1 -> Out1/1
  Ramp3/1 -> Sum5/3  "Wind Disturbance"

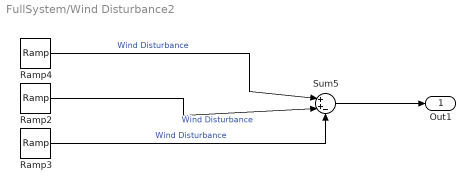
== system FullSystem/Wind Disturbance2 ==
  Ramp2 : simulink/Sources/Ramp  slope=1  start=1000  InitialOutput=0
  Ramp3 : simulink/Sources/Ramp  slope=2  start=1005  InitialOutput=0
  Ramp4 : simulink/Sources/Ramp  slope=1  start=1010  InitialOutput=0
  Sum5 : Sum  Inputs=|++-
  Out1 : Outport
  wires:
  Ramp2/1 -> Sum5/2  "Wind Disturbance"
  Ramp4/1 -> Sum5/1  "Wind Disturbance"
  Sum5/1 -> Out1/1
  Ramp3/1 -> Sum5/3  "Wind Disturbance"

== system FullSystem/Wind Disturbance3 ==
  Ramp2 : simulink/Sources/Ramp  slope=1  start=1000  InitialOutput=0
  Ramp3 : simulink/Sources/Ramp  slope=2  start=1005  InitialOutput=0
  Ramp4 : simulink/Sources/Ramp  slope=1  start=1010  InitialOutput=0
  Sum5 : Sum  Inputs=|++-
  Out1 : Outport
  wires:
  Ramp2/1 -> Sum5/2  "Wind Disturbance"
  Ramp4/1 -> Sum5/1  "Wind Disturbance"
  Sum5/1 -> Out1/1
  Ramp3/1 -> Sum5/3  "Wind Disturbance"

== system FullSystem/Wind Disturbance4 ==
  Ramp2 : simulink/Sources/Ramp  slope=1  start=1000  InitialOutput=0
  Ramp3 : simulink/Sources/Ramp  slope=2  start=1005  InitialOutput=0
  Ramp4 : simulink/Sources/Ramp  slope=1  start=1010  InitialOutput=0
  Sum5 : Sum  Inputs=|++-
  Out1 : Outport
  wires:
  Ramp2/1 -> Sum5/2  "Wind Disturbance"
  Ramp4/1 -> Sum5/1  "Wind Disturbance"
  Sum5/1 -> Out1/1
  Ramp3/1 -> Sum5/3  "Wind Disturbance"

== matlab function FullSystem/Subsystem2/Non-Linear ==
  data: Beta input; MOI_NonLinear output; Mass_Panel input; Length_Panel input; Width_Panel input; Thickness_Panel input; I_Motor input; GearRatio input; I_Pole input
function MOI_NonLinear = fcn(Beta,Mass_Panel,Length_Panel,Width_Panel,Thickness_Panel,I_Motor,GearRatio,I_Pole)
MOI_NonLinear = I_Motor + GearRatio^2*((Mass_Panel/12)*(Length_Panel^2*cos(Beta)^2 + Thickness_Panel^2*sin(Beta)^2 + Width_Panel^2)+I_Pole);

== matlab function FullSystem/Subsystem2/Linear MOI ==
  data: Beta input; MOI_NonLinear output; Mass_Panel input; Length_Panel input; Width_Panel input; Thickness_Panel input; I_Pole input; I_Motor input; GearRatio input
function MOI_NonLinear = fcn(Beta,Mass_Panel,Length_Panel,Width_Panel,Thickness_Panel,I_Pole,I_Motor,GearRatio)
MOI_NonLinear = I_Motor + GearRatio^2*(((Mass_Panel/12)*(Length_Panel^2 - Length_Panel*Beta^2 + (Thickness_Panel*Beta)^2 + Width_Panel^2))+I_Pole)
